simulink model "DreiTankTest"  (R2024a)
settings: Solver=VariableStepAuto  StartTime=0.0  StopTime=inf  FixedStep=1  RelTol=1e-3
values from neighbouring files (symbols this model uses):
  A = 1    [init3TankSim.m]    (also in tankParameters.mat)
  h1init = 10    [init3TankSim.m]    (also in tankParameters.mat = 0)
  h2init = 10    [init3TankSim.m]    (also in tankParameters.mat = 0)
  h3init = 10    [init3TankSim.m]    (also in tankParameters.mat = 0)
  Ktb1to2 = 0.0334    [init3TankSim.m]    (also in tankParameters.mat)
  Ktb2to3 = 0.0334    [init3TankSim.m]    (also in tankParameters.mat)
  Kv1out = 0.02727    [init3TankSim.m]    (also in tankParameters.mat)
  Kv1to2 = 0.075    [init3TankSim.m]    (also in tankParameters.mat)
  Kv2out = 0.0045    [init3TankSim.m]    (also in tankParameters.mat)
  Kv2to3 = 0.075    [init3TankSim.m]    (also in tankParameters.mat)
  Kv3out = 0.02727    [init3TankSim.m]    (also in tankParameters.mat)
  Tube1to2onoff = 1    [init3TankSim.m]    (also in tankParameters.mat)
  Tube2to3onoff = 1    [init3TankSim.m]    (also in tankParameters.mat)
libraries: neural x23
settings Model: PacingRate=10  Creator=Pavli  LastModifiedBy=kevin

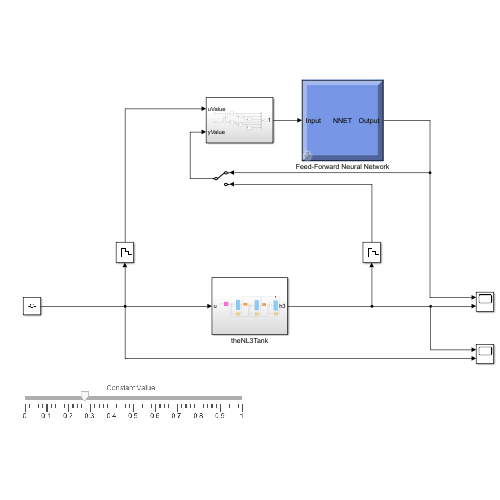
[thumbnail: Simulink's stored preview of the top-level diagram]
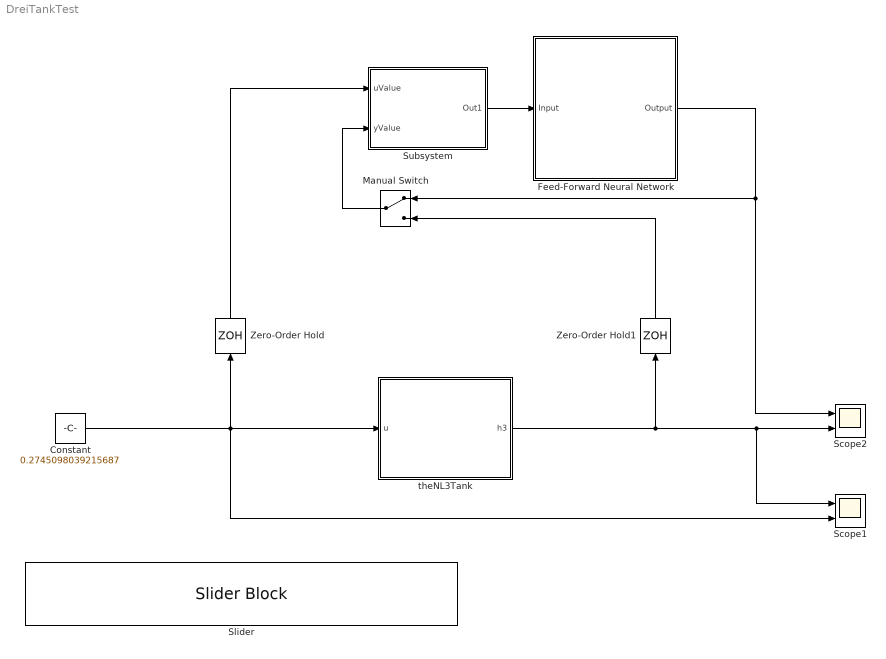
== system DreiTankTest ==
  Constant : Constant  Value=0.2745098039215687
  Feed-Forward Neural Network : Subsystem
      mask help: Feed-Forward Neural Network
      mask Display: e = 0.06;c1 = [120 150 230]/255;c2 = ([120 150 230]+0)/383;c3 = ([120 150 230]+128)/383;patch([0 1 1 0],[0 0 1 1],c1);patch([0 1 1 1-e 1-e 0+e],[0 0 1 1-e 0+e 0+e],c2);patch([0 0 1 1-e 0+e 0+e],[0 1 1 1-e 1-e 0+e],c3);plot([0 1 1 0 0],[0 0 1 1 0]);fprintf('NNET');port_label('input',1,' Input');port_label('output',1,'Output ');
  Manual Switch : ManualSwitch
  Scope1 : Scope  NumInputPorts=2
  Scope2 : Scope  NumInputPorts=2
  Slider : SliderBlock  ScaleMax=1
  Subsystem : Subsystem
  Zero-Order Hold : ZeroOrderHold
  Zero-Order Hold1 : ZeroOrderHold
  theNL3Tank : Subsystem
  wires:
  Constant/1 -> Zero-Order Hold/1, theNL3Tank/1(u), Scope1/2
  theNL3Tank/1(h3) -> Scope2/2, Scope1/1, Zero-Order Hold1/1
  Zero-Order Hold1/1 -> Manual Switch/2
  Manual Switch/1 -> Subsystem/2(yValue)
  Zero-Order Hold/1 -> Subsystem/1(uValue)
  Subsystem/1(Out1) -> Feed-Forward Neural Network/1(Input)
  Feed-Forward Neural Network/1(Output) -> Scope2/1, Manual Switch/1

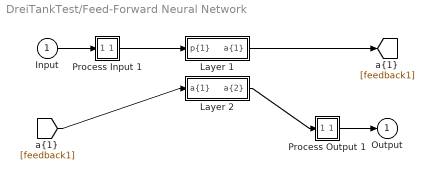
== system DreiTankTest/Feed-Forward Neural Network ==
  Input : Inport  PortDimensions=6
      mask Display: e = 0.06;c1 = [120 230 180]/255;c2 = ([120 230 180]+0)/(256+128);c3 = ([120 230 180]+128)/(256+128);patch([0 1 1 0],[0 0 1 1],c1);patch([0 1 1 1-e 1-e 0+e],[0 0 1 1-e 0+e 0+e],c2);patch([0 0 1 1-e 0+e 0+e],[0 1 1 1-e 1-e 0+e],c3);plot([0 1 1 0 0],[0 0 1 1 0]);
  Layer 1 : Subsystem
      mask Display: e = 0.06;c1 = [120 150 230]/255;c2 = ([120 150 230]+0)/383;c3 = ([120 150 230]+128)/383;patch([0 1 1 0],[0 0 1 1],c1);patch([0 1 1 1-e 1-e 0+e],[0 0 1 1-e 0+e 0+e],c2);patch([0 0 1 1-e 0+e 0+e],[0 1 1 1-e 1-e 0+e],c3);plot([0 1 1 0 0],[0 0 1 1 0]);
  Layer 2 : Subsystem
      mask Display: e = 0.06;c1 = [120 150 230]/255;c2 = ([120 150 230]+0)/383;c3 = ([120 150 230]+128)/383;patch([0 1 1 0],[0 0 1 1],c1);patch([0 1 1 1-e 1-e 0+e],[0 0 1 1-e 0+e 0+e],c2);patch([0 0 1 1-e 0+e 0+e],[0 1 1 1-e 1-e 0+e],c3);plot([0 1 1 0 0],[0 0 1 1 0]);
  Process Input 1 : Subsystem
      mask Display: e = 0.06;c1 = [120 150 230]/255;c2 = ([120 150 230]+0)/383;c3 = ([120 150 230]+128)/383;patch([0 1 1 0],[0 0 1 1],c1);patch([0 1 1 1-e 1-e 0+e],[0 0 1 1-e 0+e 0+e],c2);patch([0 0 1 1-e 0+e 0+e],[0 1 1 1-e 1-e 0+e],c3);plot([0 1 1 0 0],[0 0 1 1 0]);
  Process Output 1 : Subsystem
      mask Display: e = 0.06;c1 = [120 150 230]/255;c2 = ([120 150 230]+0)/383;c3 = ([120 150 230]+128)/383;patch([0 1 1 0],[0 0 1 1],c1);patch([0 1 1 1-e 1-e 0+e],[0 0 1 1-e 0+e 0+e],c2);patch([0 0 1 1-e 0+e 0+e],[0 1 1 1-e 1-e 0+e],c3);plot([0 1 1 0 0],[0 0 1 1 0]);
  Output : Outport  InitialOutput=0
      mask Display: e = 0.06;c1 = [120 230 180]/255;c2 = ([120 230 180]+0)/(256+128);c3 = ([120 230 180]+128)/(256+128);patch([0 1 1 0],[0 0 1 1],c1);patch([0 1 1 1-e 1-e 0+e],[0 0 1 1-e 0+e 0+e],c2);patch([0 0 1 1-e 0+e 0+e],[0 1 1 1-e 1-e 0+e],c3);plot([0 1 1 0 0],[0 0 1 1 0]);
  wires:
  Input/1 -> Process Input 1/1(x)
  Process Output 1/1(y) -> Output/1
  Process Input 1/1(p) -> Layer 1/1("p{1}")
  Layer 1/1("a{1}") -> [feedback1]
  [feedback1] -> Layer 2/1("a{1} ")
  Layer 2/1("a{2}") -> Process Output 1/1(a)

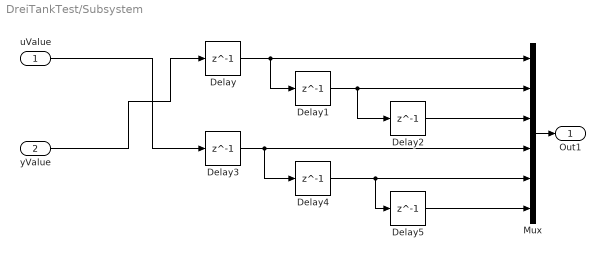
== system DreiTankTest/Subsystem ==
  uValue : Inport
  yValue : Inport  Port=2
  Delay{,1..5} (6 alike) : Delay  DelayLength=1  InitialCondition=0
  Mux : Mux  Inputs=6
  Out1 : Outport
  wires:
  Delay/1 -> Delay1/1, Mux/1
  Delay1/1 -> Delay2/1, Mux/2
  Mux/1 -> Out1/1
  uValue/1 -> Delay3/1
  Delay2/1 -> Mux/3
  yValue/1 -> Delay/1
  Delay3/1 -> Delay4/1, Mux/4
  Delay4/1 -> Delay5/1, Mux/5
  Delay5/1 -> Mux/6

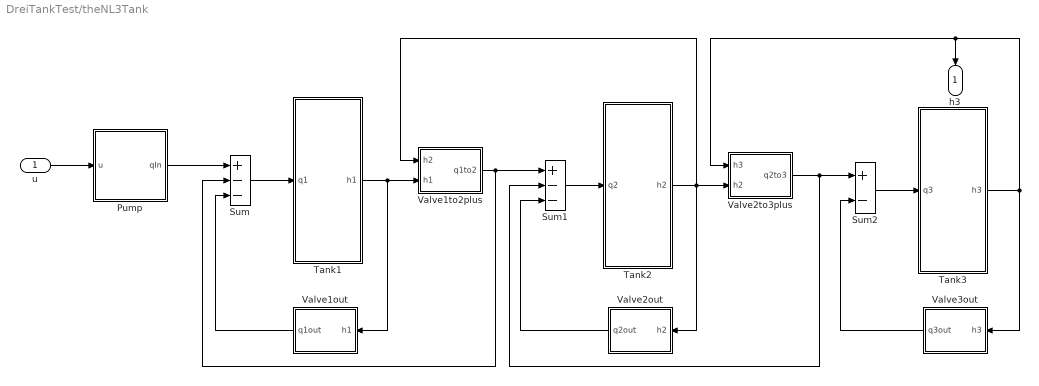
== system DreiTankTest/theNL3Tank ==
  u : Inport
  Pump : Subsystem
  Sum : Sum  Inputs=+--
  Sum1 : Sum  Inputs=+--
  Sum2 : Sum  Inputs=+-
  Tank1 : Subsystem
  Tank2 : Subsystem
  Tank3 : Subsystem
  Valve1out : Subsystem
  Valve1to2plus : Subsystem
  Valve2out : Subsystem
  Valve2to3plus : Subsystem
  Valve3out : Subsystem
  h3 : Outport
  wires:
  u/1 -> Pump/1(u)
  Tank1/1(h1) -> Valve1out/1(h1), Valve1to2plus/2(h1)
  Tank2/1(h2) -> Valve2to3plus/2(h2), Valve1to2plus/1(h2), Valve2out/1(h2)
  Valve1to2plus/1(q1to2) -> Sum1/1, Sum/2
  Valve2out/1(q2out) -> Sum1/3
  Valve1out/1(q1out) -> Sum/3
  Valve3out/1(q3out) -> Sum2/2
  Tank3/1(h3) -> Valve2to3plus/1(h3), h3/1, Valve3out/1(h3)
  Valve2to3plus/1(q2to3) -> Sum2/1, Sum1/2
  Pump/1(qIn) -> Sum/1
  Sum1/1 -> Tank2/1(q2)
  Sum2/1 -> Tank3/1(q3)
  Sum/1 -> Tank1/1(q1)

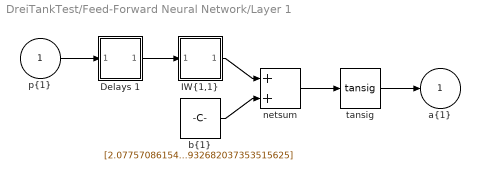
== system DreiTankTest/Feed-Forward Neural Network/Layer 1 ==
  "p{1}" : Inport  PortDimensions=6
      mask Display: e = 0.06;c1 = [120 230 180]/255;c2 = ([120 230 180]+0)/(256+128);c3 = ([120 230 180]+128)/(256+128);patch([0 1 1 0],[0 0 1 1],c1);patch([0 1 1 1-e 1-e 0+e],[0 0 1 1-e 0+e 0+e],c2);patch([0 0 1 1-e 0+e 0+e],[0 1 1 1-e 1-e 0+e],c3);plot([0 1 1 0 0],[0 0 1 1 0]);
  Delays 1 : Subsystem
      mask Display: e = 0.06;c1 = [120 150 230]/255;c2 = ([120 150 230]+0)/383;c3 = ([120 150 230]+128)/383;patch([0 1 1 0],[0 0 1 1],c1);patch([0 1 1 1-e 1-e 0+e],[0 0 1 1-e 0+e 0+e],c2);patch([0 0 1 1-e 0+e 0+e],[0 1 1 1-e 1-e 0+e],c3);plot([0 1 1 0 0],[0 0 1 1 0]);disp('0');
  "IW{1,1}" : Subsystem
      mask Display: e = 0.06;c1 = [120 150 230]/255;c2 = ([120 150 230]+0)/383;c3 = ([120 150 230]+128)/383;patch([0 1 1 0],[0 0 1 1],c1);patch([0 1 1 1-e 1-e 0+e],[0 0 1 1-e 0+e 0+e],c2);patch([0 0 1 1-e 0+e 0+e],[0 1 1 1-e 1-e 0+e],c3);plot([0 1 1 0 0],[0 0 1 1 0]);disp('W');
  "b{1}" : Constant  Value=[2.077570861542060054460989704239182174205780029296875;1.98331026691500422742819864652119576930999755859375;2.571842912830004213020629322272725403308868408203125;-1.417613371154293755438402513391338288784027099609375;-1.5166195639426949259842558603850193321704864501953125;1.0156026285300405742617613213951699435710906982421875;0.322029795376373162429928243000176735222339630126953125;0.29917391513224067534082450947607867419719696044921875;-0.09975516278283659554748652453781687654554843902587890625;-0.1298049643488832505244801041044411249458789825439453125;0.41125586209925157898936731726280413568019866943359375;0.5823449040756276673391766962595283985137939453125;0.75801806789565528976737596167367883026599884033203125;1.2580265843946374371142837844672612845897674560546875;-1.4893999945777753879383453750051558017730712890625;1.086721138460007285431174750556237995624542236328125;1.888003099909706161696476556244306266307830810546875;1.99990754623613753437894047237932682037353515625]
      mask Display: e = 0.06;c1 = [120 150 230]/255;c2 = ([120 150 230]+0)/383;c3 = ([120 150 230]+128)/383;patch([0 1 1 0],[0 0 1 1],c1);patch([0 1 1 1-e 1-e 0+e],[0 0 1 1-e 0+e 0+e],c2);patch([0 0 1 1-e 0+e 0+e],[0 1 1 1-e 1-e 0+e],c3);plot([0 1 1 0 0],[0 0 1 1 0]);disp('b');
  netsum : Sum  Inputs=2  InputSameDT=on  SaturateOnIntegerOverflow=on  OutDataTypeStr=Inherit: Same as first input
      mask Display: e = 0.06;c1 = [120 150 230]/255;c2 = ([120 150 230]+0)/383;c3 = ([120 150 230]+128)/383;patch([0 1 1 0],[0 0 1 1],c1);patch([0 1 1 1-e 1-e 0+e],[0 0 1 1-e 0+e 0+e],c2);patch([0 0 1 1-e 0+e 0+e],[0 1 1 1-e 1-e 0+e],c3);plot([0 1 1 0 0],[0 0 1 1 0]);disp('+');
  tansig : neural/Transfer Functions/tansig
  "a{1}" : Outport  InitialOutput=[0;0;0;0;0;0;0;0;0;0;0;0;0;0;0;0;0;0]
      mask Display: e = 0.06;c1 = [120 230 180]/255;c2 = ([120 230 180]+0)/(256+128);c3 = ([120 230 180]+128)/(256+128);patch([0 1 1 0],[0 0 1 1],c1);patch([0 1 1 1-e 1-e 0+e],[0 0 1 1-e 0+e 0+e],c2);patch([0 0 1 1-e 0+e 0+e],[0 1 1 1-e 1-e 0+e],c3);plot([0 1 1 0 0],[0 0 1 1 0]);
  wires:
  "p{1}"/1 -> Delays 1/1("p{1}")
  Delays 1/1("pd{1,1}") -> "IW{1,1}"/1("pd{1,1}")
  "IW{1,1}"/1("iz{1,1}") -> netsum/1
  "b{1}"/1 -> netsum/2
  netsum/1 -> tansig/1
  tansig/1 -> "a{1}"/1

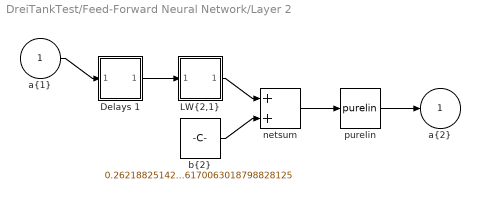
== system DreiTankTest/Feed-Forward Neural Network/Layer 2 ==
  "a{1} " : Inport  PortDimensions=18
      mask Display: e = 0.06;c1 = [120 230 180]/255;c2 = ([120 230 180]+0)/(256+128);c3 = ([120 230 180]+128)/(256+128);patch([0 1 1 0],[0 0 1 1],c1);patch([0 1 1 1-e 1-e 0+e],[0 0 1 1-e 0+e 0+e],c2);patch([0 0 1 1-e 0+e 0+e],[0 1 1 1-e 1-e 0+e],c3);plot([0 1 1 0 0],[0 0 1 1 0]);
  Delays 1 : Subsystem
      mask Display: e = 0.06;c1 = [120 150 230]/255;c2 = ([120 150 230]+0)/383;c3 = ([120 150 230]+128)/383;patch([0 1 1 0],[0 0 1 1],c1);patch([0 1 1 1-e 1-e 0+e],[0 0 1 1-e 0+e 0+e],c2);patch([0 0 1 1-e 0+e 0+e],[0 1 1 1-e 1-e 0+e],c3);plot([0 1 1 0 0],[0 0 1 1 0]);disp('0');
  "LW{2,1}" : Subsystem
      mask Display: e = 0.06;c1 = [120 150 230]/255;c2 = ([120 150 230]+0)/383;c3 = ([120 150 230]+128)/383;patch([0 1 1 0],[0 0 1 1],c1);patch([0 1 1 1-e 1-e 0+e],[0 0 1 1-e 0+e 0+e],c2);patch([0 0 1 1-e 0+e 0+e],[0 1 1 1-e 1-e 0+e],c3);plot([0 1 1 0 0],[0 0 1 1 0]);disp('W');
  "b{2}" : Constant  Value=0.262188251423154827790540366549976170063018798828125
      mask Display: e = 0.06;c1 = [120 150 230]/255;c2 = ([120 150 230]+0)/383;c3 = ([120 150 230]+128)/383;patch([0 1 1 0],[0 0 1 1],c1);patch([0 1 1 1-e 1-e 0+e],[0 0 1 1-e 0+e 0+e],c2);patch([0 0 1 1-e 0+e 0+e],[0 1 1 1-e 1-e 0+e],c3);plot([0 1 1 0 0],[0 0 1 1 0]);disp('b');
  netsum : Sum  Inputs=2  InputSameDT=on  SaturateOnIntegerOverflow=on  OutDataTypeStr=Inherit: Same as first input
      mask Display: e = 0.06;c1 = [120 150 230]/255;c2 = ([120 150 230]+0)/383;c3 = ([120 150 230]+128)/383;patch([0 1 1 0],[0 0 1 1],c1);patch([0 1 1 1-e 1-e 0+e],[0 0 1 1-e 0+e 0+e],c2);patch([0 0 1 1-e 0+e 0+e],[0 1 1 1-e 1-e 0+e],c3);plot([0 1 1 0 0],[0 0 1 1 0]);disp('+');
  purelin : neural/Transfer Functions/purelin
  "a{2}" : Outport  InitialOutput=0
      mask Display: e = 0.06;c1 = [120 230 180]/255;c2 = ([120 230 180]+0)/(256+128);c3 = ([120 230 180]+128)/(256+128);patch([0 1 1 0],[0 0 1 1],c1);patch([0 1 1 1-e 1-e 0+e],[0 0 1 1-e 0+e 0+e],c2);patch([0 0 1 1-e 0+e 0+e],[0 1 1 1-e 1-e 0+e],c3);plot([0 1 1 0 0],[0 0 1 1 0]);
  wires:
  "a{1} "/1 -> Delays 1/1("p{2}")
  Delays 1/1("pd{2,1}") -> "LW{2,1}"/1("ad{2,1}")
  "LW{2,1}"/1("lz{2,1}") -> netsum/1
  "b{2}"/1 -> netsum/2
  netsum/1 -> purelin/1
  purelin/1 -> "a{2}"/1

== system DreiTankTest/Feed-Forward Neural Network/Process Input 1 ==
  x : Inport  PortDimensions=6
      mask Display: e = 0.06;c1 = [120 230 180]/255;c2 = ([120 230 180]+0)/(256+128);c3 = ([120 230 180]+128)/(256+128);patch([0 1 1 0],[0 0 1 1],c1);patch([0 1 1 1-e 1-e 0+e],[0 0 1 1-e 0+e 0+e],c2);patch([0 0 1 1-e 0+e 0+e],[0 1 1 1-e 1-e 0+e],c3);plot([0 1 1 0 0],[0 0 1 1 0]);
  mapminmax : neural/Processing Functions/mapminmax  xmin=[0;0;0;0.00183766960512143917583216534695;0.00183766960512143917583216534695;0.00183766960512143917583216534695]  xmax=[82.2950323461710695482906885445;82.2950323461710695482906885445;82.2950323461710695482906885445;0.998998080361762408330150719848;0.998998080361762408330150719848;0.998998080361762408330150719848]  ymin=-1  ymax=1
  p : Outport  PortDimensions=6
      mask Display: e = 0.06;c1 = [120 230 180]/255;c2 = ([120 230 180]+0)/(256+128);c3 = ([120 230 180]+128)/(256+128);patch([0 1 1 0],[0 0 1 1],c1);patch([0 1 1 1-e 1-e 0+e],[0 0 1 1-e 0+e 0+e],c2);patch([0 0 1 1-e 0+e 0+e],[0 1 1 1-e 1-e 0+e],c3);plot([0 1 1 0 0],[0 0 1 1 0]);
  wires:
  x/1 -> mapminmax/1
  mapminmax/1 -> p/1

== system DreiTankTest/Feed-Forward Neural Network/Process Output 1 ==
  a : Inport  PortDimensions=1
      mask Display: e = 0.06;c1 = [120 230 180]/255;c2 = ([120 230 180]+0)/(256+128);c3 = ([120 230 180]+128)/(256+128);patch([0 1 1 0],[0 0 1 1],c1);patch([0 1 1 1-e 1-e 0+e],[0 0 1 1-e 0+e 0+e],c2);patch([0 0 1 1-e 0+e 0+e],[0 1 1 1-e 1-e 0+e],c3);plot([0 1 1 0 0],[0 0 1 1 0]);
  mapminmax_reverse : neural/Processing Functions/mapminmax_reverse  xmin=0  xmax=82.2950323461710695482906885445  ymin=-1  ymax=1
  y : Outport  PortDimensions=1
      mask Display: e = 0.06;c1 = [120 230 180]/255;c2 = ([120 230 180]+0)/(256+128);c3 = ([120 230 180]+128)/(256+128);patch([0 1 1 0],[0 0 1 1],c1);patch([0 1 1 1-e 1-e 0+e],[0 0 1 1-e 0+e 0+e],c2);patch([0 0 1 1-e 0+e 0+e],[0 1 1 1-e 1-e 0+e],c3);plot([0 1 1 0 0],[0 0 1 1 0]);
  wires:
  a/1 -> mapminmax_reverse/1
  mapminmax_reverse/1 -> y/1

== system DreiTankTest/theNL3Tank/Pump ==
  u : Inport
  InflowOrOutflowPump : Switch  Criteria=u2 > Threshold  SaturateOnIntegerOverflow=off  InputSameDT=off
  qIn : Outport
  wires:
  u/1 -> InflowOrOutflowPump/1, InflowOrOutflowPump/3, InflowOrOutflowPump/2
  InflowOrOutflowPump/1 -> qIn/1

== system DreiTankTest/theNL3Tank/Tank1 ==
  q1 : Inport
  0to100percent : Integrator  InitialConditionSource=external  LimitOutput=on  UpperSaturationLimit=100  LowerSaturationLimit=0
  Constant : Constant  Value=h1init
  Gain : Gain  Gain=1/A
  h1 : Outport
  wires:
  0to100percent/1 -> h1/1
  Gain/1 -> 0to100percent/1
  Constant/1 -> 0to100percent/2
  q1/1 -> Gain/1

== system DreiTankTest/theNL3Tank/Tank2 ==
  q2 : Inport
  0to100percent : Integrator  InitialConditionSource=external  LimitOutput=on  UpperSaturationLimit=100  LowerSaturationLimit=0
  Constant : Constant  Value=h2init
  Gain : Gain  Gain=1/A
  h2 : Outport
  wires:
  Constant/1 -> 0to100percent/2
  Gain/1 -> 0to100percent/1
  0to100percent/1 -> h2/1
  q2/1 -> Gain/1

== system DreiTankTest/theNL3Tank/Tank3 ==
  q3 : Inport
  0to100percent : Integrator  InitialConditionSource=external  LimitOutput=on  UpperSaturationLimit=100  LowerSaturationLimit=0
  Constant : Constant  Value=h3init
  Gain : Gain  Gain=1/A
  h3 : Outport
  wires:
  q3/1 -> Gain/1
  Constant/1 -> 0to100percent/2
  Gain/1 -> 0to100percent/1
  0to100percent/1 -> h3/1

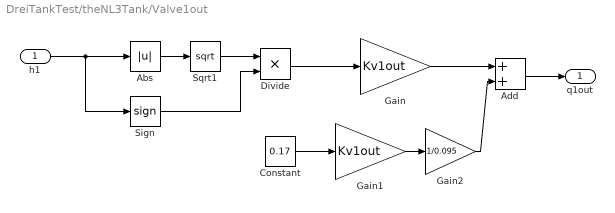
== system DreiTankTest/theNL3Tank/Valve1out ==
  h1 : Inport
  Abs : Abs  SaturateOnIntegerOverflow=off
  Add : Sum
  Constant : Constant  Value=0.17
  Divide : Product
  Gain : Gain  Gain=Kv1out
  Gain1 : Gain  Gain=Kv1out
  Gain2 : Gain  Gain=1/0.095
  Sign : Signum
  Sqrt1 : Sqrt
  q1out : Outport
  wires:
  Sqrt1/1 -> Divide/1
  Sign/1 -> Divide/2
  h1/1 -> Sign/1, Abs/1
  Abs/1 -> Sqrt1/1
  Gain/1 -> Add/1
  Add/1 -> q1out/1
  Gain1/1 -> Gain2/1
  Gain2/1 -> Add/2
  Constant/1 -> Gain1/1
  Divide/1 -> Gain/1

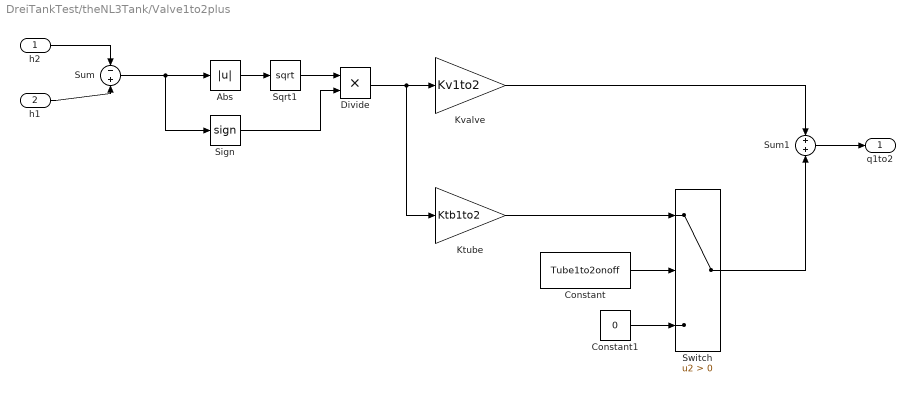
== system DreiTankTest/theNL3Tank/Valve1to2plus ==
  h2 : Inport
  h1 : Inport  Port=2
  Abs : Abs  SaturateOnIntegerOverflow=off
  Constant : Constant  Value=Tube1to2onoff
  Constant1 : Constant  Value=0
  Divide : Product
  Ktube : Gain  Gain=Ktb1to2
  Kvalve : Gain  Gain=Kv1to2
  Sign : Signum
  Sqrt1 : Sqrt
  Sum : Sum  Inputs=-+
  Sum1 : Sum
  Switch : Switch  Criteria=u2 > Threshold  SaturateOnIntegerOverflow=off  InputSameDT=off
  q1to2 : Outport
  wires:
  h1/1 -> Sum/2
  h2/1 -> Sum/1
  Sum/1 -> Sign/1, Abs/1
  Kvalve/1 -> Sum1/1
  Sum1/1 -> q1to2/1
  Divide/1 -> Ktube/1, Kvalve/1
  Switch/1 -> Sum1/2
  Constant/1 -> Switch/2
  Ktube/1 -> Switch/1
  Constant1/1 -> Switch/3
  Abs/1 -> Sqrt1/1
  Sqrt1/1 -> Divide/1
  Sign/1 -> Divide/2

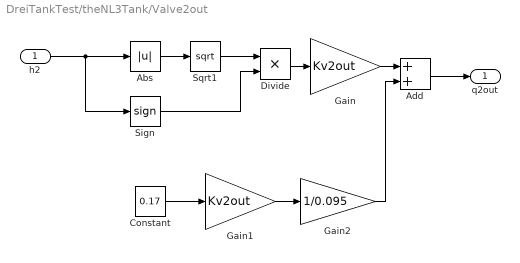
== system DreiTankTest/theNL3Tank/Valve2out ==
  h2 : Inport
  Abs : Abs  SaturateOnIntegerOverflow=off
  Add : Sum
  Constant : Constant  Value=0.17
  Divide : Product
  Gain : Gain  Gain=Kv2out
  Gain1 : Gain  Gain=Kv2out
  Gain2 : Gain  Gain=1/0.095
  Sign : Signum
  Sqrt1 : Sqrt
  q2out : Outport
  wires:
  Divide/1 -> Gain/1
  Sqrt1/1 -> Divide/1
  Sign/1 -> Divide/2
  h2/1 -> Sign/1, Abs/1
  Abs/1 -> Sqrt1/1
  Gain2/1 -> Add/2
  Gain/1 -> Add/1
  Add/1 -> q2out/1
  Constant/1 -> Gain1/1
  Gain1/1 -> Gain2/1

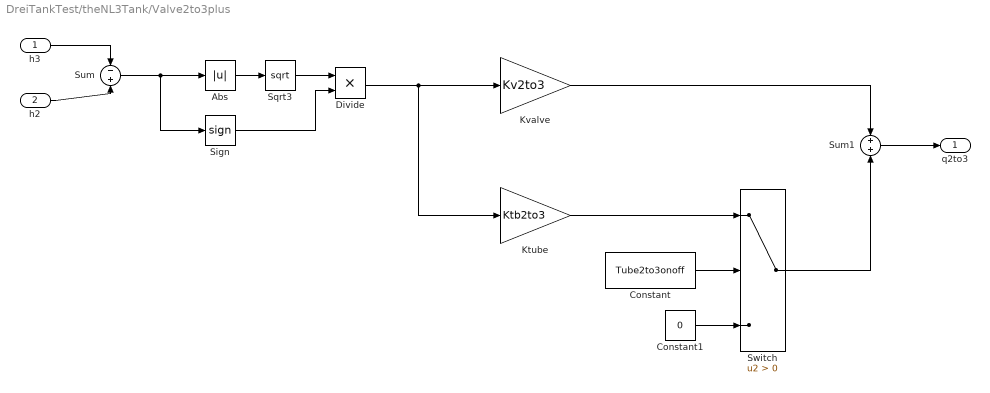
== system DreiTankTest/theNL3Tank/Valve2to3plus ==
  h3 : Inport
  h2 : Inport  Port=2
  Abs : Abs  SaturateOnIntegerOverflow=off
  Constant : Constant  Value=Tube2to3onoff
  Constant1 : Constant  Value=0
  Divide : Product
  Ktube : Gain  Gain=Ktb2to3
  Kvalve : Gain  Gain=Kv2to3
  Sign : Signum
  Sqrt3 : Sqrt
  Sum : Sum  Inputs=-+
  Sum1 : Sum
  Switch : Switch  Criteria=u2 > Threshold  SaturateOnIntegerOverflow=off  InputSameDT=off
  q2to3 : Outport
  wires:
  Sum1/1 -> q2to3/1
  Kvalve/1 -> Sum1/1
  Ktube/1 -> Switch/1
  Constant1/1 -> Switch/3
  Divide/1 -> Ktube/1, Kvalve/1
  Switch/1 -> Sum1/2
  Constant/1 -> Switch/2
  h2/1 -> Sum/2
  h3/1 -> Sum/1
  Sqrt3/1 -> Divide/1
  Sign/1 -> Divide/2
  Sum/1 -> Sign/1, Abs/1
  Abs/1 -> Sqrt3/1

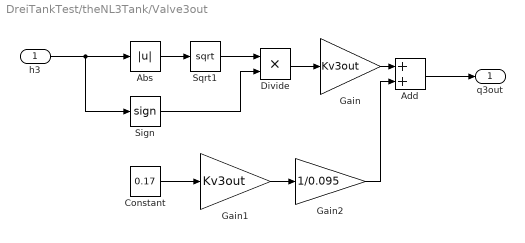
== system DreiTankTest/theNL3Tank/Valve3out ==
  h3 : Inport
  Abs : Abs  SaturateOnIntegerOverflow=off
  Add : Sum
  Constant : Constant  Value=0.17
  Divide : Product
  Gain : Gain  Gain=Kv3out
  Gain1 : Gain  Gain=Kv3out
  Gain2 : Gain  Gain=1/0.095
  Sign : Signum
  Sqrt1 : Sqrt
  q3out : Outport
  wires:
  Sqrt1/1 -> Divide/1
  Sign/1 -> Divide/2
  h3/1 -> Sign/1, Abs/1
  Abs/1 -> Sqrt1/1
  Divide/1 -> Gain/1
  Gain/1 -> Add/1
  Gain2/1 -> Add/2
  Add/1 -> q3out/1
  Gain1/1 -> Gain2/1
  Constant/1 -> Gain1/1

== system DreiTankTest/Feed-Forward Neural Network/Layer 1/Delays 1 ==
  "p{1}" : Inport  PortDimensions=6
      mask Display: e = 0.06;c1 = [120 230 180]/255;c2 = ([120 230 180]+0)/(256+128);c3 = ([120 230 180]+128)/(256+128);patch([0 1 1 0],[0 0 1 1],c1);patch([0 1 1 1-e 1-e 0+e],[0 0 1 1-e 0+e 0+e],c2);patch([0 0 1 1-e 0+e 0+e],[0 1 1 1-e 1-e 0+e],c3);plot([0 1 1 0 0],[0 0 1 1 0]);
  mux : Mux  Inputs=1
      mask Display: e = 0.06;c1 = [120 150 230]/255;c2 = ([120 150 230]+0)/383;c3 = ([120 150 230]+128)/383;patch([0 1 1 0],[0 0 1 1],c1);patch([0 1 1 1-e 1-e 0+e],[0 0 1 1-e 0+e 0+e],c2);patch([0 0 1 1-e 0+e 0+e],[0 1 1 1-e 1-e 0+e],c3);plot([0 1 1 0 0],[0 0 1 1 0]);disp('Mux')
  "pd{1,1}" : Outport
      mask Display: e = 0.06;c1 = [120 230 180]/255;c2 = ([120 230 180]+0)/(256+128);c3 = ([120 230 180]+128)/(256+128);patch([0 1 1 0],[0 0 1 1],c1);patch([0 1 1 1-e 1-e 0+e],[0 0 1 1-e 0+e 0+e],c2);patch([0 0 1 1-e 0+e 0+e],[0 1 1 1-e 1-e 0+e],c3);plot([0 1 1 0 0],[0 0 1 1 0]);
  wires:
  "p{1}"/1 -> mux/1
  mux/1 -> "pd{1,1}"/1

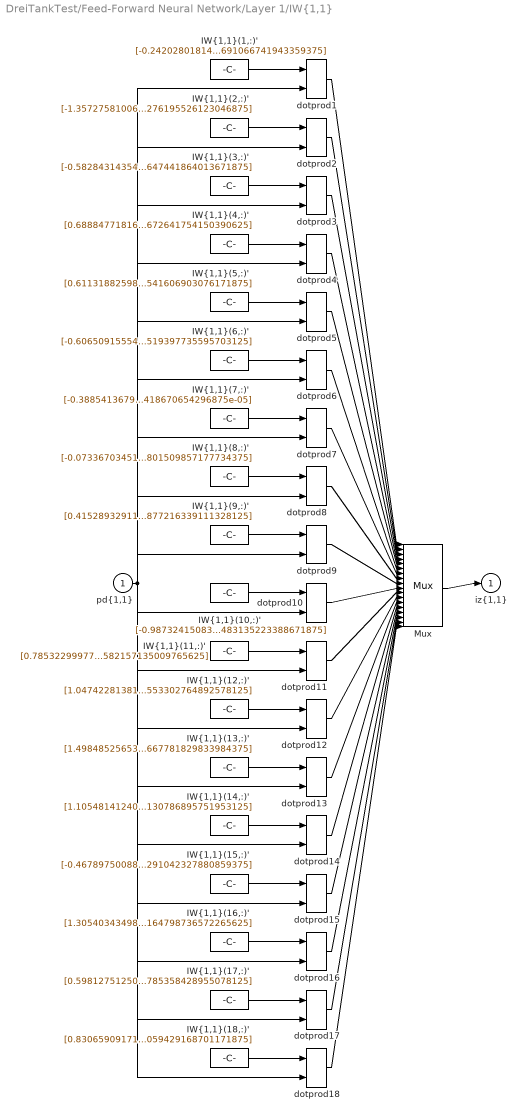
== system DreiTankTest/Feed-Forward Neural Network/Layer 1/IW{1,1} ==
  "pd{1,1}" : Inport  PortDimensions=6
      mask Display: e = 0.06;c1 = [120 230 180]/255;c2 = ([120 230 180]+0)/(256+128);c3 = ([120 230 180]+128)/(256+128);patch([0 1 1 0],[0 0 1 1],c1);patch([0 1 1 1-e 1-e 0+e],[0 0 1 1-e 0+e 0+e],c2);patch([0 0 1 1-e 0+e 0+e],[0 1 1 1-e 1-e 0+e],c3);plot([0 1 1 0 0],[0 0 1 1 0]);
  "IW{1,1}(1,:)'" : Constant  Value=[-0.2420280181476691938602385789636173285543918609619140625;0.50641321022193952483547718657064251601696014404296875;-1.1234427385709560009985352735384367406368255615234375;-1.101325845715865003882072414853610098361968994140625;1.0960969161022300344399127425276674330234527587890625;-1.350128461710281779772913068882189691066741943359375]
      mask Display: e = 0.06;c1 = [120 150 230]/255;c2 = ([120 150 230]+0)/383;c3 = ([120 150 230]+128)/383;patch([0 1 1 0],[0 0 1 1],c1);patch([0 1 1 1-e 1-e 0+e],[0 0 1 1-e 0+e 0+e],c2);patch([0 0 1 1-e 0+e 0+e],[0 1 1 1-e 1-e 0+e],c3);plot([0 1 1 0 0],[0 0 1 1 0]);disp('Weights');
  "IW{1,1}(10,:)'" : Constant  Value=[-0.98732415083121771726126780777121894061565399169921875;-0.0254688599367771661974302332964725792407989501953125;1.1624212618225941984206883716979064047336578369140625;0.57894682707193023674108189879916608333587646484375;0.07474280129399861472005994755818392150104045867919921875;-0.89638877033772501601305293661425821483135223388671875]
      mask Display: e = 0.06;c1 = [120 150 230]/255;c2 = ([120 150 230]+0)/383;c3 = ([120 150 230]+128)/383;patch([0 1 1 0],[0 0 1 1],c1);patch([0 1 1 1-e 1-e 0+e],[0 0 1 1-e 0+e 0+e],c2);patch([0 0 1 1-e 0+e 0+e],[0 1 1 1-e 1-e 0+e],c3);plot([0 1 1 0 0],[0 0 1 1 0]);disp('Weights');
  "IW{1,1}(11,:)'" : Constant  Value=[0.78532299977897401799253884746576659381389617919921875;-1.074054900759879416227704496122896671295166015625;0.866669446060435166856450450723059475421905517578125;-0.97470980633562909201117463453556410968303680419921875;1.006869616850284199216503111529164016246795654296875;-0.7733724231771808010904578623012639582157135009765625]
      mask Display: e = 0.06;c1 = [120 150 230]/255;c2 = ([120 150 230]+0)/383;c3 = ([120 150 230]+128)/383;patch([0 1 1 0],[0 0 1 1],c1);patch([0 1 1 1-e 1-e 0+e],[0 0 1 1-e 0+e 0+e],c2);patch([0 0 1 1-e 0+e 0+e],[0 1 1 1-e 1-e 0+e],c3);plot([0 1 1 0 0],[0 0 1 1 0]);disp('Weights');
  "IW{1,1}(12,:)'" : Constant  Value=[1.047422813815369835310775670222938060760498046875;-1.07283752376852259402539857546798884868621826171875;-0.30539387239825022124506403997656889259815216064453125;-0.94609638447939736760616824540193192660808563232421875;-1.096529977846170123001456886413507163524627685546875;0.77290821273386633993851546620135195553302764892578125]
      mask Display: e = 0.06;c1 = [120 150 230]/255;c2 = ([120 150 230]+0)/383;c3 = ([120 150 230]+128)/383;patch([0 1 1 0],[0 0 1 1],c1);patch([0 1 1 1-e 1-e 0+e],[0 0 1 1-e 0+e 0+e],c2);patch([0 0 1 1-e 0+e 0+e],[0 1 1 1-e 1-e 0+e],c3);plot([0 1 1 0 0],[0 0 1 1 0]);disp('Weights');
  "IW{1,1}(13,:)'" : Constant  Value=[1.4984852565349251474202674216940067708492279052734375;0.96152944373571391789567996966070495545864105224609375;0.2269708718219455023668018611715524457395076751708984375;1.25170396421588581148398588993586599826812744140625;-0.52092698623210254016413500721682794392108917236328125;-0.63111531543861276727369613581686280667781829833984375]
      mask Display: e = 0.06;c1 = [120 150 230]/255;c2 = ([120 150 230]+0)/383;c3 = ([120 150 230]+128)/383;patch([0 1 1 0],[0 0 1 1],c1);patch([0 1 1 1-e 1-e 0+e],[0 0 1 1-e 0+e 0+e],c2);patch([0 0 1 1-e 0+e 0+e],[0 1 1 1-e 1-e 0+e],c3);plot([0 1 1 0 0],[0 0 1 1 0]);disp('Weights');
  "IW{1,1}(14,:)'" : Constant  Value=[1.10548141240694075548844921286217868328094482421875;-1.0240576626525150771840344532392919063568115234375;1.0874116709333574437579272853326983749866485595703125;-0.2887226243174516593370526607031933963298797607421875;1.1737885591636600945975033027934841811656951904296875;0.6675071750165362249873624023166485130786895751953125]
      mask Display: e = 0.06;c1 = [120 150 230]/255;c2 = ([120 150 230]+0)/383;c3 = ([120 150 230]+128)/383;patch([0 1 1 0],[0 0 1 1],c1);patch([0 1 1 1-e 1-e 0+e],[0 0 1 1-e 0+e 0+e],c2);patch([0 0 1 1-e 0+e 0+e],[0 1 1 1-e 1-e 0+e],c3);plot([0 1 1 0 0],[0 0 1 1 0]);disp('Weights');
  "IW{1,1}(15,:)'" : Constant  Value=[-0.467897500888748874015021783634438179433345794677734375;-0.261793318984756384626422232031472958624362945556640625;0.388505959117106558498022650383063592016696929931640625;-0.391766881308728276422925773658789694309234619140625;1.143660680495621750907275782083161175251007080078125;1.757012812405390089764978256425820291042327880859375]
      mask Display: e = 0.06;c1 = [120 150 230]/255;c2 = ([120 150 230]+0)/383;c3 = ([120 150 230]+128)/383;patch([0 1 1 0],[0 0 1 1],c1);patch([0 1 1 1-e 1-e 0+e],[0 0 1 1-e 0+e 0+e],c2);patch([0 0 1 1-e 0+e 0+e],[0 1 1 1-e 1-e 0+e],c3);plot([0 1 1 0 0],[0 0 1 1 0]);disp('Weights');
  "IW{1,1}(16,:)'" : Constant  Value=[1.305403434989279798372763252700679004192352294921875;-1.2215432367691880788385105915949679911136627197265625;0.40160255516978560219598648473038338124752044677734375;-0.0004802545274026984449718125080863728726399131119251251220703125;0.000683674000872841187807782414864732345449738204479217529296875;-0.0004396841548952256880679334560824145228252746164798736572265625]
      mask Display: e = 0.06;c1 = [120 150 230]/255;c2 = ([120 150 230]+0)/383;c3 = ([120 150 230]+128)/383;patch([0 1 1 0],[0 0 1 1],c1);patch([0 1 1 1-e 1-e 0+e],[0 0 1 1-e 0+e 0+e],c2);patch([0 0 1 1-e 0+e 0+e],[0 1 1 1-e 1-e 0+e],c3);plot([0 1 1 0 0],[0 0 1 1 0]);disp('Weights');
  "IW{1,1}(17,:)'" : Constant  Value=[0.5981275125019649419044753813068382441997528076171875;0.990365310528500852882416438660584390163421630859375;1.1200887415450466733091161586344242095947265625;-0.838928664455638628538736156770028173923492431640625;0.1630123173454624818656810703032533638179302215576171875;-1.1370938384374646989982693412457592785358428955078125]
      mask Display: e = 0.06;c1 = [120 150 230]/255;c2 = ([120 150 230]+0)/383;c3 = ([120 150 230]+128)/383;patch([0 1 1 0],[0 0 1 1],c1);patch([0 1 1 1-e 1-e 0+e],[0 0 1 1-e 0+e 0+e],c2);patch([0 0 1 1-e 0+e 0+e],[0 1 1 1-e 1-e 0+e],c3);plot([0 1 1 0 0],[0 0 1 1 0]);disp('Weights');
  "IW{1,1}(18,:)'" : Constant  Value=[0.83065909171955876200144075482967309653759002685546875;0.365166740920840948714243268113932572305202484130859375;0.78303891898437727459025836651562713086605072021484375;0.7977734075997588991668862945516593754291534423828125;-1.0756362545492017535053719257120974361896514892578125;0.72089973705867904651967137397150509059429168701171875]
      mask Display: e = 0.06;c1 = [120 150 230]/255;c2 = ([120 150 230]+0)/383;c3 = ([120 150 230]+128)/383;patch([0 1 1 0],[0 0 1 1],c1);patch([0 1 1 1-e 1-e 0+e],[0 0 1 1-e 0+e 0+e],c2);patch([0 0 1 1-e 0+e 0+e],[0 1 1 1-e 1-e 0+e],c3);plot([0 1 1 0 0],[0 0 1 1 0]);disp('Weights');
  "IW{1,1}(2,:)'" : Constant  Value=[-1.3572758100642474676789106524665839970111846923828125;0.24173564832295946214202331248088739812374114990234375;-0.77734264760317073328366177520365454256534576416015625;-1.438251753876170990764649104676209390163421630859375;0.414797613218213234720366244800970889627933502197265625;0.177072460111006246830100963052245788276195526123046875]
      mask Display: e = 0.06;c1 = [120 150 230]/255;c2 = ([120 150 230]+0)/383;c3 = ([120 150 230]+128)/383;patch([0 1 1 0],[0 0 1 1],c1);patch([0 1 1 1-e 1-e 0+e],[0 0 1 1-e 0+e 0+e],c2);patch([0 0 1 1-e 0+e 0+e],[0 1 1 1-e 1-e 0+e],c3);plot([0 1 1 0 0],[0 0 1 1 0]);disp('Weights');
  "IW{1,1}(3,:)'" : Constant  Value=[-0.58284314354583788286845447146333754062652587890625;-0.2404352981296598301685918386283447034657001495361328125;-0.99457544430747446551066559550235979259014129638671875;-0.013230128410970189156703469279818818904459476470947265625;0.01338072585145962285768650446016181376762688159942626953125;-0.0028242381227964424676712962281044383416883647441864013671875]
      mask Display: e = 0.06;c1 = [120 150 230]/255;c2 = ([120 150 230]+0)/383;c3 = ([120 150 230]+128)/383;patch([0 1 1 0],[0 0 1 1],c1);patch([0 1 1 1-e 1-e 0+e],[0 0 1 1-e 0+e 0+e],c2);patch([0 0 1 1-e 0+e 0+e],[0 1 1 1-e 1-e 0+e],c3);plot([0 1 1 0 0],[0 0 1 1 0]);disp('Weights');
  "IW{1,1}(4,:)'" : Constant  Value=[0.68884771816582546222207383834756910800933837890625;-1.0434346560826026628632234860560856759548187255859375;-0.0336384966836004994927833422480034641921520233154296875;-1.1873903204340157113705345182097516953945159912109375;0.857247587818018796923524860176257789134979248046875;1.185262290929069539657803034060634672641754150390625]
      mask Display: e = 0.06;c1 = [120 150 230]/255;c2 = ([120 150 230]+0)/383;c3 = ([120 150 230]+128)/383;patch([0 1 1 0],[0 0 1 1],c1);patch([0 1 1 1-e 1-e 0+e],[0 0 1 1-e 0+e 0+e],c2);patch([0 0 1 1-e 0+e 0+e],[0 1 1 1-e 1-e 0+e],c3);plot([0 1 1 0 0],[0 0 1 1 0]);disp('Weights');
  "IW{1,1}(5,:)'" : Constant  Value=[0.61131882598931597261326942316372878849506378173828125;1.115200792556825692969368901685811579227447509765625;-0.8303176893568540162249291824991814792156219482421875;0.62112631571979248779058480067760683596134185791015625;-0.955325574388748322007813840173184871673583984375;0.65879561094898420048338039123336784541606903076171875]
      mask Display: e = 0.06;c1 = [120 150 230]/255;c2 = ([120 150 230]+0)/383;c3 = ([120 150 230]+128)/383;patch([0 1 1 0],[0 0 1 1],c1);patch([0 1 1 1-e 1-e 0+e],[0 0 1 1-e 0+e 0+e],c2);patch([0 0 1 1-e 0+e 0+e],[0 1 1 1-e 1-e 0+e],c3);plot([0 1 1 0 0],[0 0 1 1 0]);disp('Weights');
  "IW{1,1}(6,:)'" : Constant  Value=[-0.60650915554569284626751368705299682915210723876953125;1.4027352853893837458798543593729846179485321044921875;-0.94023810460869750027512736778589896857738494873046875;0.82751865180462369497860208866768516600131988525390625;0.58281257899498728480836007292964495718479156494140625;0.65077791246492833199255301224184222519397735595703125]
      mask Display: e = 0.06;c1 = [120 150 230]/255;c2 = ([120 150 230]+0)/383;c3 = ([120 150 230]+128)/383;patch([0 1 1 0],[0 0 1 1],c1);patch([0 1 1 1-e 1-e 0+e],[0 0 1 1-e 0+e 0+e],c2);patch([0 0 1 1-e 0+e 0+e],[0 1 1 1-e 1-e 0+e],c3);plot([0 1 1 0 0],[0 0 1 1 0]);disp('Weights');
  "IW{1,1}(7,:)'" : Constant  Value=[-0.388541367936638570856899832506314851343631744384765625;-0.0344257337282196929084676639831741340458393096923828125;0.1534225022489925371882435456427629105746746063232421875;-3.68117438341425588592924211805978984557441435754299163818359375e-05;3.8800643055758796671518562337865887457155622541904449462890625e-05;-2.38727694827942394924062685657162319330382160842418670654296875e-05]
      mask Display: e = 0.06;c1 = [120 150 230]/255;c2 = ([120 150 230]+0)/383;c3 = ([120 150 230]+128)/383;patch([0 1 1 0],[0 0 1 1],c1);patch([0 1 1 1-e 1-e 0+e],[0 0 1 1-e 0+e 0+e],c2);patch([0 0 1 1-e 0+e 0+e],[0 1 1 1-e 1-e 0+e],c3);plot([0 1 1 0 0],[0 0 1 1 0]);disp('Weights');
  "IW{1,1}(8,:)'" : Constant  Value=[-0.07336703451381042240253549380213371478021144866943359375;0.1579165421247520073588788136476068757474422454833984375;-1.836992863496672345746674182009883224964141845703125;0.40432743200279330775259722940973006188869476318359375;-0.480457086409255273995455581825808621942996978759765625;1.4286823637168077905101881697191856801509857177734375]
      mask Display: e = 0.06;c1 = [120 150 230]/255;c2 = ([120 150 230]+0)/383;c3 = ([120 150 230]+128)/383;patch([0 1 1 0],[0 0 1 1],c1);patch([0 1 1 1-e 1-e 0+e],[0 0 1 1-e 0+e 0+e],c2);patch([0 0 1 1-e 0+e 0+e],[0 1 1 1-e 1-e 0+e],c3);plot([0 1 1 0 0],[0 0 1 1 0]);disp('Weights');
  "IW{1,1}(9,:)'" : Constant  Value=[0.41528932911047167220175424517947249114513397216796875;-1.5999335074164251491168897700845263898372650146484375;0.58381332342811032010132521463674493134021759033203125;-0.4987920378076344807283248883322812616825103759765625;-0.438195867711508257880126393501996062695980072021484375;-0.993521955220530106345222520758397877216339111328125]
      mask Display: e = 0.06;c1 = [120 150 230]/255;c2 = ([120 150 230]+0)/383;c3 = ([120 150 230]+128)/383;patch([0 1 1 0],[0 0 1 1],c1);patch([0 1 1 1-e 1-e 0+e],[0 0 1 1-e 0+e 0+e],c2);patch([0 0 1 1-e 0+e 0+e],[0 1 1 1-e 1-e 0+e],c3);plot([0 1 1 0 0],[0 0 1 1 0]);disp('Weights');
  Mux : Mux  Inputs=18
      mask Display: e = 0.06;c1 = [120 150 230]/255;c2 = ([120 150 230]+0)/383;c3 = ([120 150 230]+128)/383;patch([0 1 1 0],[0 0 1 1],c1);patch([0 1 1 1-e 1-e 0+e],[0 0 1 1-e 0+e 0+e],c2);patch([0 0 1 1-e 0+e 0+e],[0 1 1 1-e 1-e 0+e],c3);plot([0 1 1 0 0],[0 0 1 1 0]);disp('Mux');
  dotprod{1..18} (18 alike) : neural/Weight Functions/dotprod
  "iz{1,1}" : Outport
      mask Display: e = 0.06;c1 = [120 230 180]/255;c2 = ([120 230 180]+0)/(256+128);c3 = ([120 230 180]+128)/(256+128);patch([0 1 1 0],[0 0 1 1],c1);patch([0 1 1 1-e 1-e 0+e],[0 0 1 1-e 0+e 0+e],c2);patch([0 0 1 1-e 0+e 0+e],[0 1 1 1-e 1-e 0+e],c3);plot([0 1 1 0 0],[0 0 1 1 0]);
  wires:
  "IW{1,1}(1,:)'"/1 -> dotprod1/1
  "pd{1,1}"/1 -> dotprod1/2, dotprod2/2, dotprod3/2, dotprod4/2, dotprod5/2, dotprod6/2, dotprod7/2, dotprod8/2, dotprod9/2, dotprod10/2, dotprod11/2, dotprod12/2, dotprod13/2, dotprod14/2, dotprod15/2, dotprod16/2, dotprod17/2, dotprod18/2
  dotprod1/1 -> Mux/1
  "IW{1,1}(2,:)'"/1 -> dotprod2/1
  dotprod2/1 -> Mux/2
  "IW{1,1}(3,:)'"/1 -> dotprod3/1
  dotprod3/1 -> Mux/3
  "IW{1,1}(4,:)'"/1 -> dotprod4/1
  dotprod4/1 -> Mux/4
  "IW{1,1}(5,:)'"/1 -> dotprod5/1
  dotprod5/1 -> Mux/5
  "IW{1,1}(6,:)'"/1 -> dotprod6/1
  dotprod6/1 -> Mux/6
  "IW{1,1}(7,:)'"/1 -> dotprod7/1
  dotprod7/1 -> Mux/7
  "IW{1,1}(8,:)'"/1 -> dotprod8/1
  dotprod8/1 -> Mux/8
  "IW{1,1}(9,:)'"/1 -> dotprod9/1
  dotprod9/1 -> Mux/9
  "IW{1,1}(10,:)'"/1 -> dotprod10/1
  dotprod10/1 -> Mux/10
  "IW{1,1}(11,:)'"/1 -> dotprod11/1
  dotprod11/1 -> Mux/11
  "IW{1,1}(12,:)'"/1 -> dotprod12/1
  dotprod12/1 -> Mux/12
  "IW{1,1}(13,:)'"/1 -> dotprod13/1
  dotprod13/1 -> Mux/13
  "IW{1,1}(14,:)'"/1 -> dotprod14/1
  dotprod14/1 -> Mux/14
  "IW{1,1}(15,:)'"/1 -> dotprod15/1
  dotprod15/1 -> Mux/15
  "IW{1,1}(16,:)'"/1 -> dotprod16/1
  dotprod16/1 -> Mux/16
  "IW{1,1}(17,:)'"/1 -> dotprod17/1
  dotprod17/1 -> Mux/17
  "IW{1,1}(18,:)'"/1 -> dotprod18/1
  dotprod18/1 -> Mux/18
  Mux/1 -> "iz{1,1}"/1

== system DreiTankTest/Feed-Forward Neural Network/Layer 2/Delays 1 ==
  "p{2}" : Inport  PortDimensions=18
      mask Display: e = 0.06;c1 = [120 230 180]/255;c2 = ([120 230 180]+0)/(256+128);c3 = ([120 230 180]+128)/(256+128);patch([0 1 1 0],[0 0 1 1],c1);patch([0 1 1 1-e 1-e 0+e],[0 0 1 1-e 0+e 0+e],c2);patch([0 0 1 1-e 0+e 0+e],[0 1 1 1-e 1-e 0+e],c3);plot([0 1 1 0 0],[0 0 1 1 0]);
  mux : Mux  Inputs=1
      mask Display: e = 0.06;c1 = [120 150 230]/255;c2 = ([120 150 230]+0)/383;c3 = ([120 150 230]+128)/383;patch([0 1 1 0],[0 0 1 1],c1);patch([0 1 1 1-e 1-e 0+e],[0 0 1 1-e 0+e 0+e],c2);patch([0 0 1 1-e 0+e 0+e],[0 1 1 1-e 1-e 0+e],c3);plot([0 1 1 0 0],[0 0 1 1 0]);disp('Mux')
  "pd{2,1}" : Outport
      mask Display: e = 0.06;c1 = [120 230 180]/255;c2 = ([120 230 180]+0)/(256+128);c3 = ([120 230 180]+128)/(256+128);patch([0 1 1 0],[0 0 1 1],c1);patch([0 1 1 1-e 1-e 0+e],[0 0 1 1-e 0+e 0+e],c2);patch([0 0 1 1-e 0+e 0+e],[0 1 1 1-e 1-e 0+e],c3);plot([0 1 1 0 0],[0 0 1 1 0]);
  wires:
  "p{2}"/1 -> mux/1
  mux/1 -> "pd{2,1}"/1

== system DreiTankTest/Feed-Forward Neural Network/Layer 2/LW{2,1} ==
  "ad{2,1}" : Inport  PortDimensions=18
      mask Display: e = 0.06;c1 = [120 230 180]/255;c2 = ([120 230 180]+0)/(256+128);c3 = ([120 230 180]+128)/(256+128);patch([0 1 1 0],[0 0 1 1],c1);patch([0 1 1 1-e 1-e 0+e],[0 0 1 1-e 0+e 0+e],c2);patch([0 0 1 1-e 0+e 0+e],[0 1 1 1-e 1-e 0+e],c3);plot([0 1 1 0 0],[0 0 1 1 0]);
  "IW{2,1}(1,:)'" : Constant  Value=[0.00017070288857823118396084272063717435230500996112823486328125;-0.000114604943253432761348688251334948517978773452341556549072265625;-0.01602230263177807645380568146720179356634616851806640625;0.000107847568705977695457075282714498598579666577279567718505859375;-7.3195713303384626695867465340228363857022486627101898193359375e-05;4.0139096152799143797716523163199298096515121869742870330810546875e-06;-3.366790218536403589411065695458091795444488525390625;-1.760744568022891052248846133210236075683496892452239990234375e-05;1.552242873545103951237085493364276089778286404907703399658203125e-05;-0.00019556630132316153562223315365287135136895813047885894775390625;-9.2665883310819597271958125705992870280169881880283355712890625e-05;2.34816093516866975800770622750945904044783674180507659912109375e-05;0.00024098984597565022906622000942178374316426925361156463623046875;1.316701027015500753756908902669664485074463300406932830810546875e-05;-2.6841399465053415654476501144010125443628567154519259929656982421875e-07;1.0073124474585497534206979253212921321392059326171875;-5.7503259567818685348895325903928466004799702204763889312744140625e-06;0.00019463949103669763557832028677552216322510503232479095458984375]
      mask Display: e = 0.06;c1 = [120 150 230]/255;c2 = ([120 150 230]+0)/383;c3 = ([120 150 230]+128)/383;patch([0 1 1 0],[0 0 1 1],c1);patch([0 1 1 1-e 1-e 0+e],[0 0 1 1-e 0+e 0+e],c2);patch([0 0 1 1-e 0+e 0+e],[0 1 1 1-e 1-e 0+e],c3);plot([0 1 1 0 0],[0 0 1 1 0]);disp('weights');
  Mux : Mux  Inputs=1
      mask Display: e = 0.06;c1 = [120 150 230]/255;c2 = ([120 150 230]+0)/383;c3 = ([120 150 230]+128)/383;patch([0 1 1 0],[0 0 1 1],c1);patch([0 1 1 1-e 1-e 0+e],[0 0 1 1-e 0+e 0+e],c2);patch([0 0 1 1-e 0+e 0+e],[0 1 1 1-e 1-e 0+e],c3);plot([0 1 1 0 0],[0 0 1 1 0]);disp('Mux');
  dotprod1 : neural/Weight Functions/dotprod
  "lz{2,1}" : Outport
      mask Display: e = 0.06;c1 = [120 230 180]/255;c2 = ([120 230 180]+0)/(256+128);c3 = ([120 230 180]+128)/(256+128);patch([0 1 1 0],[0 0 1 1],c1);patch([0 1 1 1-e 1-e 0+e],[0 0 1 1-e 0+e 0+e],c2);patch([0 0 1 1-e 0+e 0+e],[0 1 1 1-e 1-e 0+e],c3);plot([0 1 1 0 0],[0 0 1 1 0]);
  wires:
  "IW{2,1}(1,:)'"/1 -> dotprod1/1
  "ad{2,1}"/1 -> dotprod1/2
  dotprod1/1 -> Mux/1
  Mux/1 -> "lz{2,1}"/1
